simulink model "rate_limited_systems_exercise"  (R2021a)
settings: Solver=VariableStepAuto  StartTime=0.0  StopTime=25  RelTol=1e-3
values from neighbouring files (symbols this model uses):
  K_P = 1/abs(freqresp(G_ol,omega_c))    [Anti_windup_example.m]    (also in P_Lead_Lag.m = 1/abs(freqresp(G_ol,omega_c*1i)); Rate_limited_example.m; Rate_limited_exercise.m)
undefined symbols (not defined in the file or in its folder): den_D, den_PI, num_D, num_PI
settings Model: Creator=dimpa  LastModifiedBy=dimpa

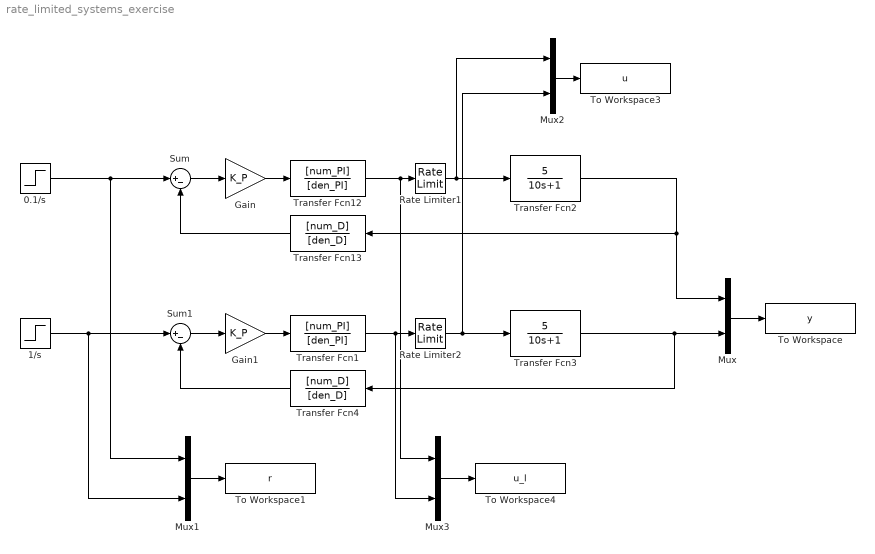
== system rate_limited_systems_exercise ==
  0.1/s : Step  After=0.1  SampleTime=0
  1/s : Step  SampleTime=0
  Gain : Gain  Gain=K_P
  Gain1 : Gain  Gain=K_P
  Mux{,1..3} (4 alike) : Mux  Inputs=2
  Rate Limiter1 : RateLimiter  SampleTimeMode=inherited
  Rate Limiter2 : RateLimiter  SampleTimeMode=inherited
  Sum : Sum  Inputs=|+-
  Sum1 : Sum  Inputs=|+-
  To Workspace : ToWorkspace  VariableName=y  SaveFormat=Timeseries  SampleTime=-1
  To Workspace1 : ToWorkspace  VariableName=r  SaveFormat=Timeseries  SampleTime=-1
  To Workspace3 : ToWorkspace  VariableName=u  SaveFormat=Timeseries  SampleTime=-1
  To Workspace4 : ToWorkspace  VariableName=u_l  SaveFormat=Timeseries  SampleTime=-1
  Transfer Fcn1 : TransferFcn  Numerator=[num_PI]  Denominator=[den_PI]
  Transfer Fcn12 : TransferFcn  Numerator=[num_PI]  Denominator=[den_PI]
  Transfer Fcn13 : TransferFcn  Numerator=[num_D]  Denominator=[den_D]
  Transfer Fcn2 : TransferFcn  Numerator=[5]  Denominator=[10 1]
  Transfer Fcn3 : TransferFcn  Numerator=[5]  Denominator=[10 1]
  Transfer Fcn4 : TransferFcn  Numerator=[num_D]  Denominator=[den_D]
  wires:
  0.1/s/1 -> Mux1/1, Sum/1
  1/s/1 -> Mux1/2, Sum1/1
  Rate Limiter1/1 -> Transfer Fcn2/1, Mux2/1
  Transfer Fcn3/1 -> Mux/2, Transfer Fcn4/1
  Transfer Fcn2/1 -> Mux/1, Transfer Fcn13/1
  Mux/1 -> To Workspace/1
  Mux1/1 -> To Workspace1/1
  Sum/1 -> Gain/1
  Gain/1 -> Transfer Fcn12/1
  Transfer Fcn12/1 -> Mux3/1, Rate Limiter1/1
  Transfer Fcn13/1 -> Sum/2
  Transfer Fcn4/1 -> Sum1/2
  Transfer Fcn1/1 -> Mux3/2, Rate Limiter2/1
  Gain1/1 -> Transfer Fcn1/1
  Sum1/1 -> Gain1/1
  Rate Limiter2/1 -> Transfer Fcn3/1, Mux2/2
  Mux2/1 -> To Workspace3/1
  Mux3/1 -> To Workspace4/1
